simulink model "productModel"  (R2015a)
settings: Solver=ode45  StartTime=0.0  StopTime=300  RelTol=1e-3
values from neighbouring files (symbols this model uses):
  alpha_const = 0.0    (= 0)    [averagedRelayOutput.m]    (also in bursting_linearised.m = 0.1; fastSlow.m; manParamsNullclines.m; manipulateParameters.m = getappdata(hObject.Parent,'alpha_const'))
  beta = 0.37    [averagedRelayOutput.m]    (also in bursting_linearised.m = 0.27; compareApproximations.m = 1.5; fastSlow.m; fast_nullcline_winged_cusp.m = 0.5)
  gamma = 0    [averagedRelayOutput.m]    (also in bursting_linearised.m = 1; compareApproximations.m = 1; fastSlow.m; fast_nullcline_winged_cusp.m = 1)
  slow_plant_X0 = -1.0    (= -1)    [averagedRelayOutput.m]    (also in bursting_linearised.m = -1.05; fastSlow.m; fast_nullcline_winged_cusp.m = -2; hRose.m = -10)
  ts = 1    [averagedRelayOutput.m]    (also in bursting_linearised.m; compareApproximations.m; fastSlow.m; fast_nullcline_winged_cusp.m)
  tus = 800    [averagedRelayOutput.m]    (also in bursting_linearised.m; fastSlow.m; manParamsNullclines.m; manipulateParameters.m = getappdata(hObject.Parent,'tus'))
settings Model: Creator=ra428  LastModifiedBy=ra428

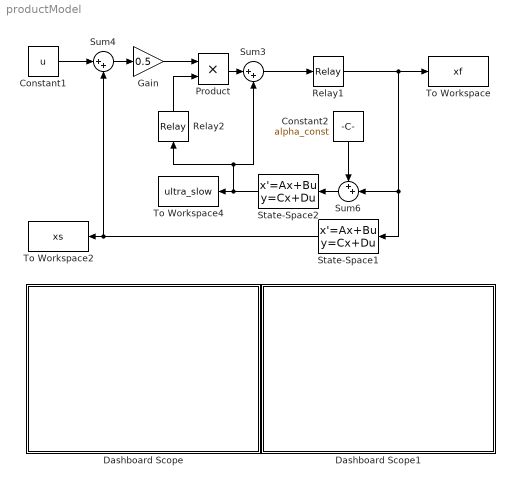
== system productModel ==
  Constant1 : Constant  Value=u
  Constant2 : Constant  Value=alpha_const
  Dashboard Scope : Subsystem  DialogController=hmiCreateDDGDialog  IsWebBlock=on  mask(MathWorksWebBlock){webBlockId=7838c4d8-368e-4e94-b7e1-c429dfe9d63f, webBlockType=sdiscope, ShowInitialText=on, HMISrcModelName=productModel}
      mask prompts: webBlockId "WebBlock Id"; webBlockType "WebBlock Type"; HMISrcModelName "Source Model"
      mask Help: helpview([docroot '/mapfiles/simulink.map'], 'hmi_scope')
      mask Display:
      | if strcmp(get_param(bdroot(gcb),'BlockDiagramType'), 'library')
      |     image([(matlabroot) '/toolbox/simulink/hmi/icons/DashboardScope.png']);
      | end
  Dashboard Scope1 : Subsystem  DialogController=hmiCreateDDGDialog  IsWebBlock=on  mask(MathWorksWebBlock){webBlockId=9d6ff472-6718-4a5f-b65c-6938d812c49a, webBlockType=sdiscope, ShowInitialText=on, HMISrcModelName=productModel}
      mask prompts: webBlockId "WebBlock Id"; webBlockType "WebBlock Type"; HMISrcModelName "Source Model"
      mask Help: helpview([docroot '/mapfiles/simulink.map'], 'hmi_scope')
      mask Display:
      | if strcmp(get_param(bdroot(gcb),'BlockDiagramType'), 'library')
      |     image([(matlabroot) '/toolbox/simulink/hmi/icons/DashboardScope.png']);
      | end
  Gain : Gain  Gain=0.5
  Product : Product
  Relay1 : Relay  OnSwitchValue=beta  OffSwitchValue=-beta  OffOutputValue=-1
  Relay2 : Relay  OnSwitchValue=beta-0.5*(u-1-0.5*gamma)  OffSwitchValue=beta  OnOutputValue=-1  OffOutputValue=1
  State-Space1 : StateSpace  A=-1/ts  B=1/ts  D=0.5*1*gamma  X0=slow_plant_X0
  State-Space2 : StateSpace  A=-1/tus  B=-1/tus  D=0  X0=0.4
  Sum3 : Sum  Inputs=|++
  Sum4 : Sum  Inputs=|++
  Sum6 : Sum  Inputs=++|
  To Workspace : ToWorkspace  VariableName=xf  SaveFormat=Timeseries  SampleTime=-1
  To Workspace2 : ToWorkspace  VariableName=xs  SaveFormat=Timeseries  SampleTime=-1
  To Workspace4 : ToWorkspace  VariableName=ultra_slow  SaveFormat=Timeseries  SampleTime=-1
  wires:
  Sum3/1 -> Relay1/1
  Constant1/1 -> Sum4/1
  Relay1/1 -> Sum6/2, State-Space1/1, To Workspace/1
  State-Space1/1 -> Sum4/2, To Workspace2/1
  Constant2/1 -> Sum6/1
  Sum6/1 -> State-Space2/1
  Sum4/1 -> Gain/1
  State-Space2/1 -> Sum3/2, Relay2/1, To Workspace4/1
  Gain/1 -> Product/1
  Product/1 -> Sum3/1
  Relay2/1 -> Product/2

== system productModel/Dashboard Scope ==

== system productModel/Dashboard Scope1 ==
